simulink model "Full Wave Thyristor"  (R2017a)
settings: Solver=VariableStepAuto  StartTime=0.0  StopTime=2  RelTol=1e-3
libraries: powerlib x11
settings Model: Creator=hp  LastModifiedBy=sujee
settings DataIOCC: ReturnWorkspaceOutputs=on
settings SFSimCC: SimUseLocalCustomCode=on
settings RTWCC: RTWUseLocalCustomCode=on

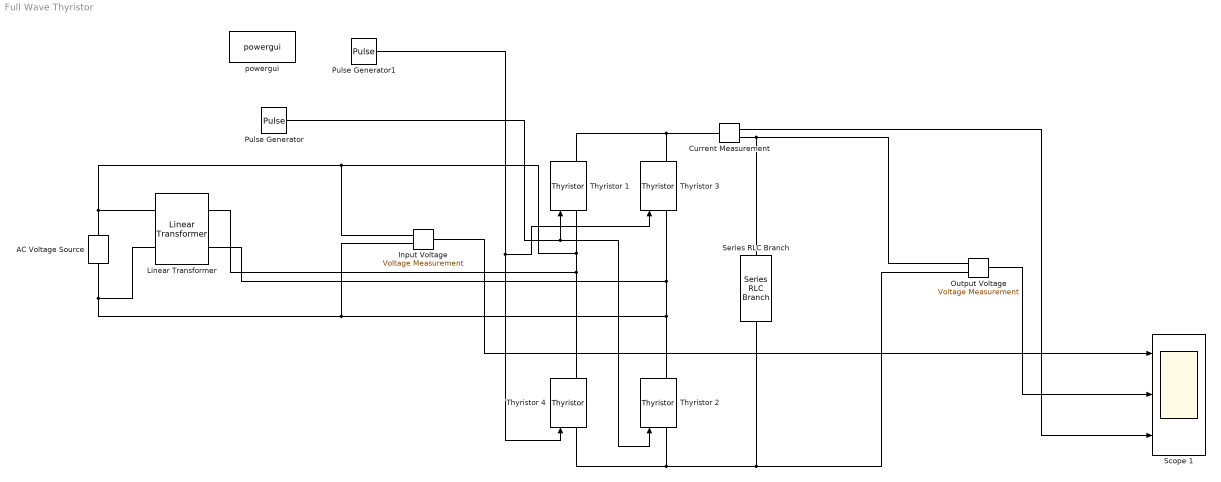
== system Full Wave Thyristor ==
  AC Voltage Source : powerlib/Electrical Sources/AC Voltage Source  Amplitude=10  Phase=0  Frequency=50  SampleTime=0  Measurements=None  BusType=swing  Pref=10e3  Qref=0  Qmin=-inf  Qmax=+inf
  Current Measurement : powerlib/Measurements/Current Measurement  PhasorSimulation=off  OutputType=Complex  PSBequivalent=0
  "Input Voltage " : powerlib/Measurements/Voltage Measurement  PhasorSimulation=off  OutputType=Complex  PSBequivalent=0
  Linear Transformer : powerlib/Elements/Linear Transformer  UNITS=pu  NominalPower=[ 250e6 60 ]  winding1="[ 735e3  0.002  0.08 ]"  winding2="[ 315e3  0.002  0.08 ]"  ThreeWindings=off  winding3="[ 315e3  0.002  0.08 ]"  RmLm=[ 500 500 ]  Measurements=None  DataType=off
  "Output Voltage " : powerlib/Measurements/Voltage Measurement  PhasorSimulation=off  OutputType=Complex  PSBequivalent=0
  Pulse Generator : DiscretePulseGenerator  PulseType=Time based  Amplitude=5  Period=0.02  PulseWidth=5  PhaseDelay=90*0.02/360
  Pulse Generator1 : DiscretePulseGenerator  PulseType=Time based  Amplitude=5  Period=0.02  PulseWidth=5  PhaseDelay=270*0.02/360
  Scope 1 : Scope  NumInputPorts=3
  Series RLC Branch : powerlib/Elements/Series RLC Branch  LConnTagsString=__new0  RConnTagsString=__new0  BranchType=R  Resistance=10  Inductance=5e-3  SetiL0=off  InitialCurrent=0  Capacitance=1e-6  Setx0=off  InitialVoltage=0  Measurements=None
  Thyristor {1..4} (4 alike) : powerlib/Power Electronics/Thyristor  Ron=0.001  Lon=0  Vf=0.8  IC=0  Rs=500  Cs=250e-9  Measurements=on
  powergui : powerlib/powergui  Priority=1  SimulationMode=Continuous  SampleTime=50e-6  frequency=60  Iterations=50  frequencyindice=50  Pbase=100e6  ErrMax=1e-4  UnitsV=kV  UnitsW=MW  buscounter=0  FunctionMessages=off  echomessages=off  EnableUseOfTLC=off  CurrentSourceSwitches=off  DisableSnubberDevices=off  DisableRonSwitches=off  DisableVfSwitches=off  DisplayEquations=off  AutomaticDiscreteSolvers=off  SolverType=Tustin/Backward Euler (TBE)  Interpol=off  ExternalGateDelay=off  methode=off  Ts=100  x0status=blocks  SPID=on  SwTol=0  HookPort=off  NonlinearTolerance=1e-4  nMaxIteration=100  ContinueOnMaxIteration=off  RestoreLinks=warning  ResistiveCurrentMeasurement=off  Frange=[0:2:500]  Ylog=off  Xlog=on  ShowGrid=off  save=off  variable=ZData  structure=0  ZoomFFT=off  StartTime=0.0  cycles=1  DisplayStyle=1  fundamental=60  FreqAxis=off  MaxFrequency=1000  frequencyindicesteady=1  RmsSteady=1  display=off
  wires:
  Pulse Generator/1 -> Thyristor 1/1, Thyristor 2/1
  Current Measurement/1 -> Scope 1/3
  "Output Voltage "/1 -> Scope 1/2
  "Input Voltage "/1 -> Scope 1/1
  Pulse Generator1/1 -> Thyristor 3/1, Thyristor 4/1
  connections:
  Thyristor 3/LConn1 -- Linear Transformer/RConn2 -- Linear Transformer/LConn2 -- AC Voltage Source/LConn1 -- "Input Voltage "/LConn2 -- Thyristor 2/RConn1
  Thyristor 1/LConn1 -- Linear Transformer/LConn1 -- AC Voltage Source/RConn1 -- "Input Voltage "/LConn1 -- Linear Transformer/RConn1 -- Thyristor 4/RConn1
  Thyristor 1/RConn1 -- Thyristor 3/RConn1 -- Current Measurement/LConn1
  Current Measurement/RConn1 -- "Output Voltage "/LConn1 -- Series RLC Branch/LConn1
  Series RLC Branch/RConn1 -- "Output Voltage "/LConn2 -- Thyristor 2/LConn1 -- Thyristor 4/LConn1
